simulink model "WindTurbine_TypeIV_HM"  (R2025a)
settings: Solver=FixedStepDiscrete  StartTime=0  StopTime=3  FixedStep=Ts  RelTol=1e-3  EnableMultiTasking=on
InitFcn:
  | load('xInitial_WPP.mat');
  | Ts = 50e-6;
undefined symbols (not defined in the file): D1, Delta, DiscIntNeverNeededParam, LowerLimit, magnitude, UpperLimit
libraries: powerlib x47, simulink x28, powerlib_meascontrol x17, powerlib_extras x6
(part 2 of 2)

== system WindTurbine_TypeIV_HM/Generic Type IV HM/Predictor4 ==
  in : Inport
  Delay : Delay  DelayLength=1  InitialCondition=Init_value  SampleTime=Ts
  Delay1 : Delay  DelayLength=1  InitialCondition=Init_value  SampleTime=Ts
  Gain : Gain  Gain=2
  Sum1 : Sum  Inputs=|+-
  out : Outport
  wires:
  Gain/1 -> Sum1/1
  Delay/1 -> Delay1/1, Gain/1
  Sum1/1 -> out/1
  Delay1/1 -> Sum1/2
  in/1 -> Delay/1

== system WindTurbine_TypeIV_HM/Generic Type IV HM/Predictor6 ==
  in : Inport
  Delay : Delay  DelayLength=1  InitialCondition=Init_value  SampleTime=Ts
  Delay1 : Delay  DelayLength=1  InitialCondition=Init_value  SampleTime=Ts
  Gain : Gain  Gain=2
  Sum1 : Sum  Inputs=|+-
  out : Outport
  wires:
  Gain/1 -> Sum1/1
  Delay/1 -> Delay1/1, Gain/1
  Sum1/1 -> out/1
  Delay1/1 -> Sum1/2
  in/1 -> Delay/1

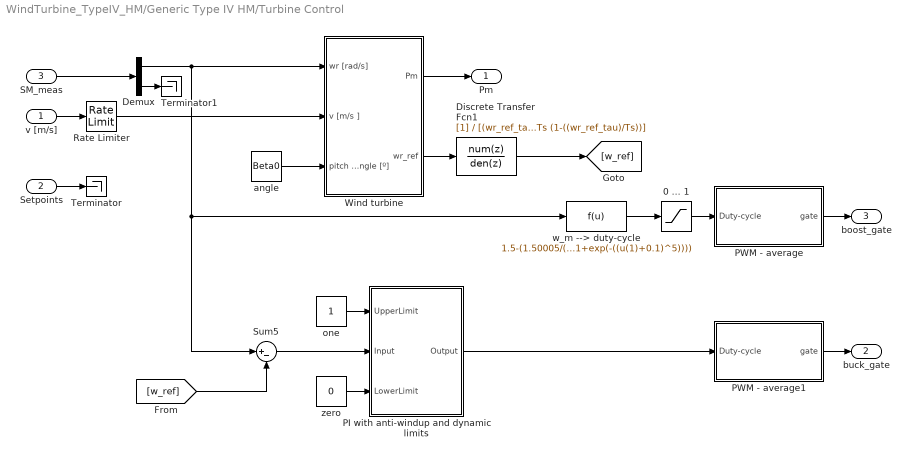
== system WindTurbine_TypeIV_HM/Generic Type IV HM/Turbine Control ==
  v [m/s] : Inport
  Setpoints : Inport  Port=2
  SM_meas : Inport  Port=3
  0 ... 1 : Saturate  UpperLimit=1  LowerLimit=0
  Demux : Demux  Outputs=2
  Discrete Transfer Fcn1 : DiscreteTransferFcn  Denominator=[(wr_ref_tau)/Ts (1-((wr_ref_tau)/Ts))]  InitialStates=w_init  SampleTime=Ts
  PI with anti-windup and dynamic limits : Subsystem  mask(Discrete PI Controller with anti-windup and dynamic limiters){Kp=Vdc1_Kp, Ki=Vdc1_Ki, Init=Vdc1_stateInit, Ts=Ts}
      mask prompts: Kp "Proportional gain (Kp):"; Ki "Integral gain (Ki):"; Init "State initial value:"; Ts "Sample time:"
      mask Display:
      | disp('PI-\nAST');
      | port_label('input',1,'UpperLimit');
      | port_label('input',2,'In');
      | port_label('input',3,'LowerLimit');
      | port_label('output',1,'Out');
  PWM - average : Subsystem  mask{fboost=f_boost, Ts=Ts}
      mask prompts: fboost "PWM frequency:"; Ts "Sample time (Ts):"
  PWM - average1 : Subsystem  mask{fboost=f_boost, Ts=Ts}
      mask prompts: fboost "PWM frequency:"; Ts "Sample time (Ts):"
  Rate Limiter : RateLimiter  RisingSlewLimit=v_rise_rate  FallingSlewLimit=v_fall_rate  SampleTimeMode=inherited  InitialCondition=v_init
  Sum5 : Sum  Inputs=|+-
  Terminator : Terminator
  Terminator1 : Terminator
  Wind turbine : Subsystem
  angle : Constant  Value=Beta0
  one : Constant
  w_m --> duty-cycle : Fcn  Expr=1.5-(1.50005/(1+exp(-((u(1)+0.1)^5))))
  zero : Constant  Value=0
  Pm : Outport
  buck_gate : Outport  Port=2
  boost_gate : Outport  Port=3
  wires:
  [w_ref] -> Sum5/2
  angle/1 -> Wind turbine/3(pitch angle [º])
  w_m --> duty-cycle/1 -> 0 ... 1/1
  0 ... 1/1 -> PWM - average/1(Duty-cycle)
  Rate Limiter/1 -> Wind turbine/2("v [m/s ] ")
  PWM - average/1(gate) -> boost_gate/1
  v [m/s]/1 -> Rate Limiter/1
  Wind turbine/1(Pm) -> Pm/1
  Wind turbine/2(wr_ref) -> Discrete Transfer Fcn1/1
  Setpoints/1 -> Terminator/1
  SM_meas/1 -> Demux/1
  Demux/1 -> w_m --> duty-cycle/1, Sum5/1, Wind turbine/1(wr [rad/s])
  Demux/2 -> Terminator1/1
  Sum5/1 -> PI with anti-windup and dynamic limits/2(Input)
  Discrete Transfer Fcn1/1 -> [w_ref]
  zero/1 -> PI with anti-windup and dynamic limits/3(LowerLimit)
  one/1 -> PI with anti-windup and dynamic limits/1(UpperLimit)
  PI with anti-windup and dynamic limits/1(Output) -> PWM - average1/1(Duty-cycle)
  PWM - average1/1(gate) -> buck_gate/1

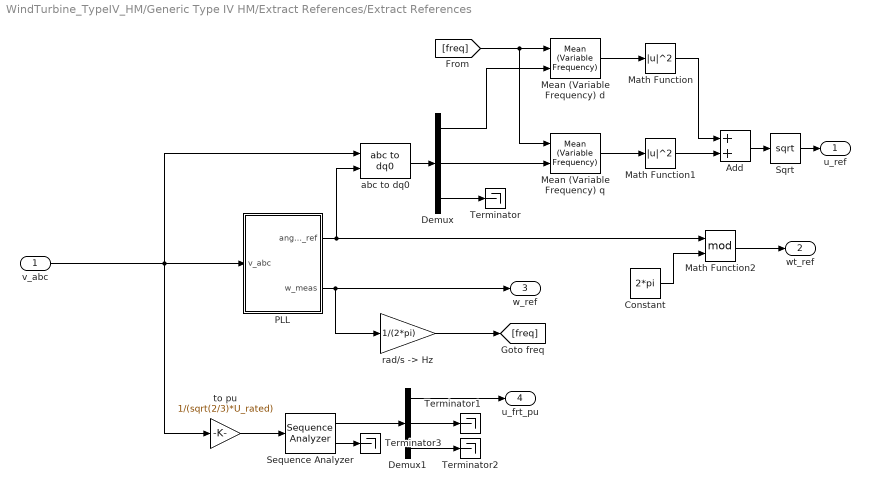
== system WindTurbine_TypeIV_HM/Generic Type IV HM/Extract References/Extract References ==
  v_abc : Inport
  Add : Sum
  Constant : Constant  Value=2*pi
  Demux : Demux  Outputs=3
  Demux1 : Demux  Outputs=3
  Math Function : Math  Operator=magnitude^2  SignedPower=on
  Math Function1 : Math  Operator=magnitude^2  SignedPower=on
  Math Function2 : Math  Operator=mod  SignedPower=on
  Mean (Variable Frequency) d : powerlib_meascontrol/Measurements/Mean (Variable Frequency)  Finit=f_rated  Fmin=0.9*f_rated  Vinit=0  Ts=Ts
  Mean (Variable Frequency) q : powerlib_meascontrol/Measurements/Mean (Variable Frequency)  Finit=f_rated  Fmin=0.9*f_rated  Vinit=0  Ts=Ts
  PLL : Subsystem
  Sequence Analyzer : powerlib_meascontrol/Measurements/Sequence Analyzer  Freq=f_rated  n=1  seq=Positive Negative Zero  InInit=[1, 0]  Ts=Ts
  Sqrt : Sqrt
  Terminator{,1..3} (4 alike) : Terminator
  abc to dq0 : powerlib_meascontrol/Transformations/abc to dq0  Alignment=90 degrees behind phase A axis
  "rad/s -> Hz" : Gain  Gain=1/(2*pi)
  to pu : Gain  Gain=1/(sqrt(2/3)*U_rated)
  u_ref : Outport
  wt_ref : Outport  Port=2
  w_ref : Outport  Port=3
  u_frt_pu : Outport  Port=4
  wires:
  abc to dq0/1 -> Demux/1
  Demux/3 -> Terminator/1
  Math Function/1 -> Add/1
  PLL/1(angle_ref) -> abc to dq0/2, Math Function2/1
  Math Function1/1 -> Add/2
  Add/1 -> Sqrt/1
  Sqrt/1 -> u_ref/1
  v_abc/1 -> PLL/1(v_abc), to pu/1, abc to dq0/1
  Sequence Analyzer/1 -> Demux1/1
  Demux1/2 -> Terminator1/1
  Demux1/3 -> Terminator2/1
  Sequence Analyzer/2 -> Terminator3/1
  Demux1/1 -> u_frt_pu/1
  [freq] -> Mean (Variable Frequency) q/1, Mean (Variable Frequency) d/1
  Mean (Variable Frequency) d/1 -> Math Function/1
  Demux/1 -> Mean (Variable Frequency) d/2
  Mean (Variable Frequency) q/1 -> Math Function1/1
  Demux/2 -> Mean (Variable Frequency) q/2
  Constant/1 -> Math Function2/2
  Math Function2/1 -> wt_ref/1
  PLL/2(w_meas) -> w_ref/1, "rad/s -> Hz"/1
  "rad/s -> Hz"/1 -> [freq]
  to pu/1 -> Sequence Analyzer/1

== system WindTurbine_TypeIV_HM/Generic Type IV HM/Extract References/Measurement Filter (Current) ==
  Meas_in : Inport
  Demux : Demux  Outputs=3
      settings: DisplayOption=none
  Discrete 2nd-Order Filter2 : powerlib_extras/Discrete  Control Blocks/Discrete  2nd-Order Filter  FilterType=Lowpass  Fo=Freq  Zeta=Zeta  Ts=Ts  Initialize=off  Vac_Init=[0.8 -25 60]  Vdc_Init=-0.4  PlotResponse=off  param1=[1 500 1]
  Discrete 2nd-Order Filter3 : powerlib_extras/Discrete  Control Blocks/Discrete  2nd-Order Filter  FilterType=Lowpass  Fo=Freq  Zeta=Zeta  Ts=Ts  Initialize=off  Vac_Init=[0.8 -25 60]  Vdc_Init=-0.4  PlotResponse=off  param1=[1 500 1]
  Discrete 2nd-Order Filter4 : powerlib_extras/Discrete  Control Blocks/Discrete  2nd-Order Filter  FilterType=Lowpass  Fo=Freq  Zeta=Zeta  Ts=Ts  Initialize=off  Vac_Init=[0.8 -25 60]  Vdc_Init=-0.4  PlotResponse=off  param1=[1 500 1]
  Mux1 : Mux  Inputs=3
  Filt_out : Outport
  wires:
  Discrete 2nd-Order Filter4/1 -> Mux1/3
  Discrete 2nd-Order Filter3/1 -> Mux1/2
  Demux/3 -> Discrete 2nd-Order Filter4/1
  Demux/1 -> Discrete 2nd-Order Filter2/1
  Meas_in/1 -> Demux/1
  Demux/2 -> Discrete 2nd-Order Filter3/1
  Discrete 2nd-Order Filter2/1 -> Mux1/1
  Mux1/1 -> Filt_out/1

== system WindTurbine_TypeIV_HM/Generic Type IV HM/Extract References/Measurement Filter (Voltage) ==
  Meas_in : Inport
  Demux : Demux  Outputs=3
      settings: DisplayOption=none
  Discrete 2nd-Order Filter2 : powerlib_extras/Discrete  Control Blocks/Discrete  2nd-Order Filter  FilterType=Lowpass  Fo=Freq  Zeta=Zeta  Ts=Ts  Initialize=off  Vac_Init=[0.8 -25 60]  Vdc_Init=-0.4  PlotResponse=off  param1=[1 500 1]
  Discrete 2nd-Order Filter3 : powerlib_extras/Discrete  Control Blocks/Discrete  2nd-Order Filter  FilterType=Lowpass  Fo=Freq  Zeta=Zeta  Ts=Ts  Initialize=off  Vac_Init=[0.8 -25 60]  Vdc_Init=-0.4  PlotResponse=off  param1=[1 500 1]
  Discrete 2nd-Order Filter4 : powerlib_extras/Discrete  Control Blocks/Discrete  2nd-Order Filter  FilterType=Lowpass  Fo=Freq  Zeta=Zeta  Ts=Ts  Initialize=off  Vac_Init=[0.8 -25 60]  Vdc_Init=-0.4  PlotResponse=off  param1=[1 500 1]
  Mux1 : Mux  Inputs=3
  Filt_out : Outport
  wires:
  Mux1/1 -> Filt_out/1
  Discrete 2nd-Order Filter2/1 -> Mux1/1
  Demux/2 -> Discrete 2nd-Order Filter3/1
  Meas_in/1 -> Demux/1
  Demux/1 -> Discrete 2nd-Order Filter2/1
  Demux/3 -> Discrete 2nd-Order Filter4/1
  Discrete 2nd-Order Filter3/1 -> Mux1/2
  Discrete 2nd-Order Filter4/1 -> Mux1/3

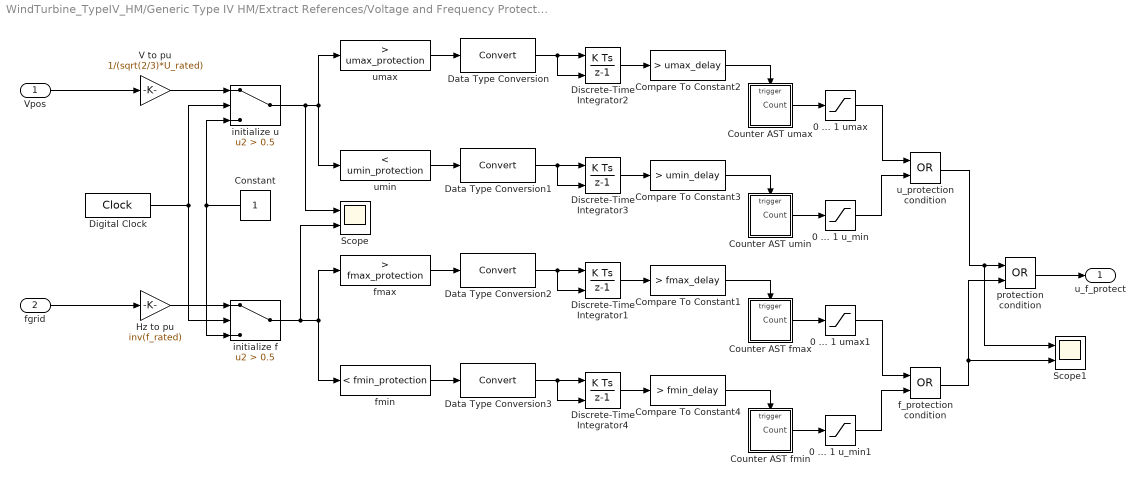
== system WindTurbine_TypeIV_HM/Generic Type IV HM/Extract References/Voltage and Frequency Protection ==
  Vpos : Inport
  fgrid : Inport  Port=2
  0 ... 1 u_min : Saturate  UpperLimit=1  LowerLimit=0
  0 ... 1 u_min1 : Saturate  UpperLimit=1  LowerLimit=0
  0 ... 1 umax : Saturate  UpperLimit=1  LowerLimit=0
  0 ... 1 umax1 : Saturate  UpperLimit=1  LowerLimit=0
  Compare To Constant1 : simulink/Logic and Bit Operations/Compare To Constant  relop=>  const=fmax_delay  OutDataTypeStr=boolean
  Compare To Constant2 : simulink/Logic and Bit Operations/Compare To Constant  relop=>  const=umax_delay  OutDataTypeStr=boolean
  Compare To Constant3 : simulink/Logic and Bit Operations/Compare To Constant  relop=>  const=umin_delay  OutDataTypeStr=boolean
  Compare To Constant4 : simulink/Logic and Bit Operations/Compare To Constant  relop=>  const=fmin_delay  OutDataTypeStr=boolean
  Constant : Constant
  Counter AST fmax : Subsystem
  Counter AST fmin : Subsystem
  Counter AST umax : Subsystem
  Counter AST umin : Subsystem
  Data Type Conversion{,1..3} (4 alike) : DataTypeConversion  SaturateOnIntegerOverflow=off  RndMeth=Floor
  Digital Clock : DigitalClock  SampleTime=Ts
  Discrete-Time Integrator{1..4} (4 alike) : DiscreteIntegrator  ExternalReset=falling  SampleTime=Ts  ICPrevOutput=DiscIntNeverNeededParam  ICPrevScaledInput=DiscIntNeverNeededParam
  Hz to pu : Gain  Gain=inv(f_rated)
  Scope : Scope  NumInputPorts=2
      settings: ActiveDisplayYMinimum=-0.20067  ActiveDisplayYMaximum=1.81542
  Scope1 : Scope  NumInputPorts=2
      settings: ActiveDisplayYMinimum=-1  ActiveDisplayYMaximum=1  DataLoggingVariableName=ScopeData2
  V to pu : Gain  Gain=1/(sqrt(2/3)*U_rated)
  f_protection condition : Logic  Operator=OR  AllPortsSameDT=off  OutDataTypeStr=boolean
  fmax : simulink/Logic and Bit Operations/Compare To Constant  relop=>  const=fmax_protection  OutDataTypeStr=boolean
  fmin : simulink/Logic and Bit Operations/Compare To Constant  relop=<  const=fmin_protection  OutDataTypeStr=boolean
  initialize f : Switch  Criteria=u2 > Threshold  Threshold=0.5  SaturateOnIntegerOverflow=off  InputSameDT=off
  initialize u : Switch  Criteria=u2 > Threshold  Threshold=0.5  SaturateOnIntegerOverflow=off  InputSameDT=off
  protection condition : Logic  Operator=OR  AllPortsSameDT=off  OutDataTypeStr=boolean
  u_protection condition : Logic  Operator=OR  AllPortsSameDT=off  OutDataTypeStr=boolean
  umax : simulink/Logic and Bit Operations/Compare To Constant  relop=>  const=umax_protection  OutDataTypeStr=boolean
  umin : simulink/Logic and Bit Operations/Compare To Constant  relop=<  const=umin_protection  OutDataTypeStr=boolean
  u_f_protect : Outport
  wires:
  Discrete-Time Integrator1/1 -> Compare To Constant1/1
  Counter AST fmin/1(Count) -> 0 ... 1 u_min1/1
  Compare To Constant4/1 -> Counter AST fmin/Trigger
  umax/1 -> Data Type Conversion/1
  0 ... 1 u_min/1 -> u_protection condition/2
  Discrete-Time Integrator3/1 -> Compare To Constant3/1
  Compare To Constant1/1 -> Counter AST fmax/Trigger
  Counter AST umin/1(Count) -> 0 ... 1 u_min/1
  fmin/1 -> Data Type Conversion3/1
  0 ... 1 umax1/1 -> f_protection condition/1
  Discrete-Time Integrator4/1 -> Compare To Constant4/1
  Counter AST fmax/1(Count) -> 0 ... 1 umax1/1
  Data Type Conversion/1 -> Discrete-Time Integrator2/2, Discrete-Time Integrator2/1
  umin/1 -> Data Type Conversion1/1
  Compare To Constant3/1 -> Counter AST umin/Trigger
  Compare To Constant2/1 -> Counter AST umax/Trigger
  fmax/1 -> Data Type Conversion2/1
  0 ... 1 u_min1/1 -> f_protection condition/2
  Data Type Conversion3/1 -> Discrete-Time Integrator4/2, Discrete-Time Integrator4/1
  Data Type Conversion2/1 -> Discrete-Time Integrator1/1, Discrete-Time Integrator1/2
  Discrete-Time Integrator2/1 -> Compare To Constant2/1
  0 ... 1 umax/1 -> u_protection condition/1
  Counter AST umax/1(Count) -> 0 ... 1 umax/1
  Data Type Conversion1/1 -> Discrete-Time Integrator3/1, Discrete-Time Integrator3/2
  fgrid/1 -> Hz to pu/1
  V to pu/1 -> initialize u/1
  Hz to pu/1 -> initialize f/1
  f_protection condition/1 -> Scope1/2, protection condition/2
  protection condition/1 -> u_f_protect/1
  Digital Clock/1 -> initialize u/2, initialize f/2
  Constant/1 -> initialize f/3, initialize u/3
  initialize u/1 -> Scope/1, umin/1, umax/1
  Vpos/1 -> V to pu/1
  u_protection condition/1 -> Scope1/1, protection condition/1
  initialize f/1 -> Scope/2, fmax/1, fmin/1

== system WindTurbine_TypeIV_HM/Generic Type IV HM/Grid-Side Inverter Control/Counter AST ==
  Trigger : TriggerPort  VariantControl=Variant  PortDimensions=1
  Constant : Constant
  Memory : Memory  InheritSampleTime=on
  Sum : Sum  Inputs=|++
  Count : Outport
  wires:
  Constant/1 -> Sum/2
  Sum/1 -> Memory/1, Count/1
  Memory/1 -> Sum/1

== system WindTurbine_TypeIV_HM/Generic Type IV HM/Grid-Side Inverter Control/FRT_ramp_p ==
  note: Aramis Schwanka Trevisan adapted from:
      | Beat Ronner
      | ABB Industrie AG
      | Turgi, Switzerland
  UpperLimit : Inport
  u : Inport  Port=2
  LowerLimit : Inport  Port=3
  Saturation : simulink/Discontinuities/Saturation Dynamic  OutMin=[]  OutMax=[]  OutDataTypeStr=Inherit: Same as second input  OutDataType=fixdt(1, 16)  OutScaling=2^-10  DoSatur=off
  Sum : Sum  Inputs=|++  InputSameDT=on  SaturateOnIntegerOverflow=on  OutDataTypeStr=Inherit: Same as first input
  Sum7 : Sum  Inputs=|+-  InputSameDT=on  SaturateOnIntegerOverflow=on  OutDataTypeStr=Inherit: Same as first input
  Unit Delay : UnitDelay  InitialCondition=1  SampleTime=Ts  HasFrameUpgradeWarning=on
  l Ts : Gain  Gain=Ts
  u Ts : Gain  Gain=Ts
  y : Outport
  wires:
  Sum7/1 -> Saturation/2
  Saturation/1 -> Sum/1
  UpperLimit/1 -> u Ts/1
  LowerLimit/1 -> l Ts/1
  Sum/1 -> Unit Delay/1, y/1  "y"
  Unit Delay/1 -> Sum/2, Sum7/2  "y-1"
  u/1 -> Sum7/1
  u Ts/1 -> Saturation/1
  l Ts/1 -> Saturation/3

== system WindTurbine_TypeIV_HM/Generic Type IV HM/Grid-Side Inverter Control/FRT_ramp_q ==
  note: Aramis Schwanka Trevisan adapted from:
      | Beat Ronner
      | ABB Industrie AG
      | Turgi, Switzerland
  UpperLimit : Inport
  u : Inport  Port=2
  LowerLimit : Inport  Port=3
  Saturation : simulink/Discontinuities/Saturation Dynamic  OutMin=[]  OutMax=[]  OutDataTypeStr=Inherit: Same as second input  OutDataType=fixdt(1, 16)  OutScaling=2^-10  DoSatur=off
  Sum : Sum  Inputs=|++  InputSameDT=on  SaturateOnIntegerOverflow=on  OutDataTypeStr=Inherit: Same as first input
  Sum7 : Sum  Inputs=|+-  InputSameDT=on  SaturateOnIntegerOverflow=on  OutDataTypeStr=Inherit: Same as first input
  Unit Delay : UnitDelay  InitialCondition=1  SampleTime=Ts  HasFrameUpgradeWarning=on
  l Ts : Gain  Gain=Ts
  u Ts : Gain  Gain=Ts
  y : Outport
  wires:
  l Ts/1 -> Saturation/3
  u Ts/1 -> Saturation/1
  u/1 -> Sum7/1
  Unit Delay/1 -> Sum7/2, Sum/2  "y-1"
  Sum/1 -> y/1, Unit Delay/1  "y"
  LowerLimit/1 -> l Ts/1
  UpperLimit/1 -> u Ts/1
  Saturation/1 -> Sum/1
  Sum7/1 -> Saturation/2

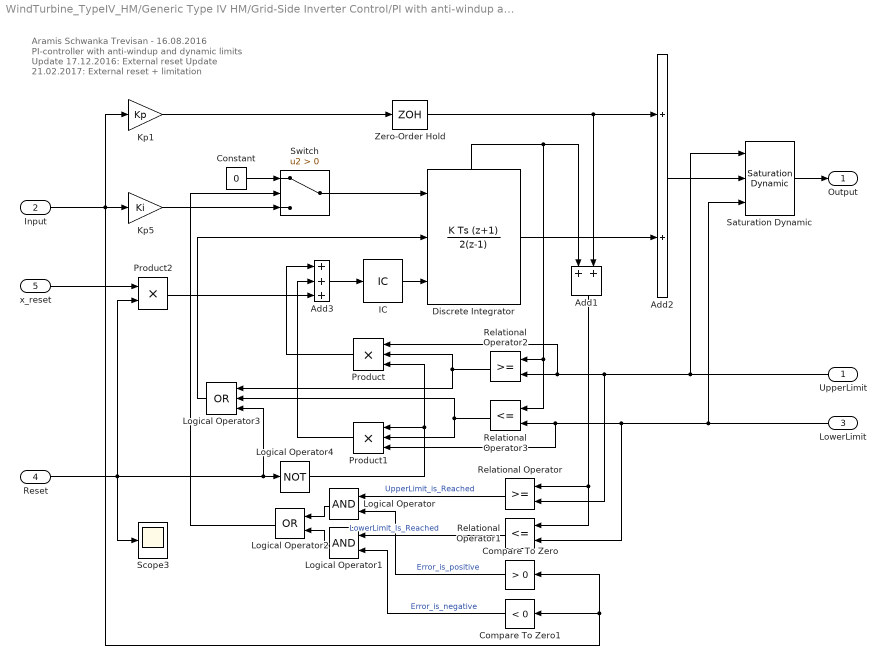
== system WindTurbine_TypeIV_HM/Generic Type IV HM/Grid-Side Inverter Control/PI with anti-windup and dynamic limits - Id ==
  note: Aramis Schwanka Trevisan - 16.08.2016
      | PI-controller with anti-windup and dynamic limits
      | Update 17.12.2016: External reset
      | Update 21.02.2017: External reset + limitation
  UpperLimit : Inport
  Input : Inport  Port=2
  LowerLimit : Inport  Port=3
  Reset : Inport  Port=4
  x_reset : Inport  Port=5
  Add1 : Sum
  Add2 : Sum
  Add3 : Sum  Inputs=+++
  Compare To Zero : simulink/Logic and Bit Operations/Compare To Zero  relop=>  OutDataTypeStr=uint8  ZeroCross=off
  Compare To Zero1 : simulink/Logic and Bit Operations/Compare To Zero  relop=<  OutDataTypeStr=uint8  ZeroCross=off
  Constant : Constant  Value=0
  Discrete Integrator : DiscreteIntegrator  IntegratorMethod=Integration: Trapezoidal  gainval=1  ExternalReset=sampled level  InitialConditionSource=external  InitialCondition=Init  SampleTime=Ts  UpperSaturationLimit=UpperLimit  LowerSaturationLimit=LowerLimit  ShowStatePort=on  ICPrevOutput=DiscIntNeverNeededParam  ICPrevScaledInput=DiscIntNeverNeededParam
  IC : InitialCondition  Value=Init
  Kp1 : Gain  Gain=Kp  SaturateOnIntegerOverflow=on  SampleTime=Ts  OutDataTypeStr=Inherit: Same as input  ParamDataTypeStr=Inherit: Same as input
  Kp5 : Gain  Gain=Ki  SaturateOnIntegerOverflow=on  SampleTime=Ts  OutDataTypeStr=Inherit: Same as input  ParamDataTypeStr=Inherit: Same as input
  Logical Operator : Logic  AllPortsSameDT=off  OutDataTypeStr=boolean
  Logical Operator1 : Logic  AllPortsSameDT=off  OutDataTypeStr=boolean
  Logical Operator2 : Logic  Operator=OR  AllPortsSameDT=off  OutDataTypeStr=boolean
  Logical Operator3 : Logic  Operator=OR  Inputs=3  AllPortsSameDT=off  OutDataTypeStr=boolean
  Logical Operator4 : Logic  Operator=NOT  Inputs=3  AllPortsSameDT=off  OutDataTypeStr=boolean
  Product : Product  Inputs=3
  Product1 : Product  Inputs=3
  Product2 : Product
  Relational Operator : RelationalOperator  OutDataTypeStr=boolean  InputSameDT=off
  Relational Operator1 : RelationalOperator  Operator=<=  OutDataTypeStr=boolean  InputSameDT=off
  Relational Operator2 : RelationalOperator  OutDataTypeStr=boolean  InputSameDT=off
  Relational Operator3 : RelationalOperator  Operator=<=  OutDataTypeStr=boolean  InputSameDT=off
  Saturation Dynamic : simulink/Discontinuities/Saturation Dynamic  OutMin=[]  OutMax=[]  OutDataTypeStr=Inherit: Same as second input  OutDataType=fixdt(1, 16)  OutScaling=2^-10  DoSatur=off
  Scope3 : Scope
      settings: ActiveDisplayYMinimum=-0.125  ActiveDisplayYMaximum=1.125
  Switch : Switch  Criteria=u2 > Threshold  SaturateOnIntegerOverflow=off  InputSameDT=off
  Zero-Order Hold : ZeroOrderHold  SampleTime=Ts
  Output : Outport
  wires:
  Reset/1 -> Scope3/1, Product2/2, Logical Operator3/3, Logical Operator4/1
  IC/1 -> Discrete Integrator/3
  Switch/1 -> Discrete Integrator/1
  Compare To Zero1/1 -> Logical Operator1/2  "Error_is_negative"
  Logical Operator/1 -> Logical Operator2/1
  Relational Operator/1 -> Logical Operator/1  "UpperLimit_is_Reached"
  Relational Operator1/1 -> Logical Operator1/1  "LowerLimit_Is_Reached"
  Saturation Dynamic/1 -> Output/1
  Logical Operator2/1 -> Switch/2
  Constant/1 -> Switch/1
  Kp5/1 -> Switch/3
  Add2/1 -> Saturation Dynamic/2
  Kp1/1 -> Zero-Order Hold/1
  Add1/1 -> Relational Operator/1, Relational Operator1/1
  Input/1 -> Kp5/1, Compare To Zero1/1, Compare To Zero/1, Kp1/1
  Compare To Zero/1 -> Logical Operator/2  "Error_is_positive"
  Logical Operator1/1 -> Logical Operator2/2
  Relational Operator2/1 -> Logical Operator3/1, Product/2
  Relational Operator3/1 -> Product1/2, Logical Operator3/2
  Logical Operator3/1 -> Discrete Integrator/2
  Add3/1 -> IC/1
  Product1/1 -> Add3/2
  UpperLimit/1 -> Saturation Dynamic/1, Relational Operator/2, Product/1, Relational Operator2/2
  Discrete Integrator/State -> Add1/1, Relational Operator3/1, Relational Operator2/1
  Discrete Integrator/1 -> Add2/2
  Logical Operator4/1 -> Product/3, Product1/1
  LowerLimit/1 -> Saturation Dynamic/3, Relational Operator1/2, Relational Operator3/2, Product1/3
  Product2/1 -> Add3/3
  Product/1 -> Add3/1
  x_reset/1 -> Product2/1
  Zero-Order Hold/1 -> Add2/1, Add1/2

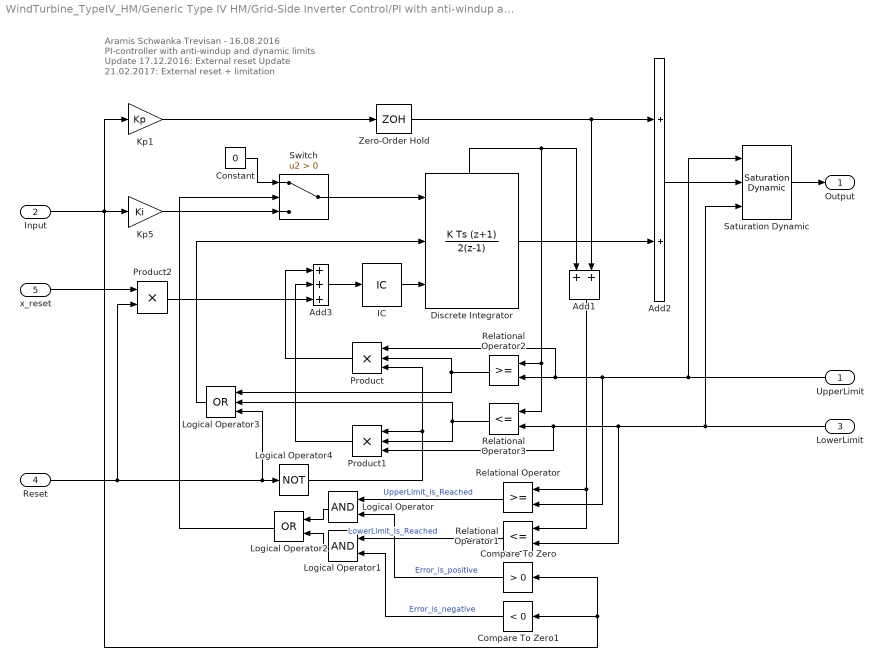
== system WindTurbine_TypeIV_HM/Generic Type IV HM/Grid-Side Inverter Control/PI with anti-windup and dynamic limits - Iq ==
  note: Aramis Schwanka Trevisan - 16.08.2016
      | PI-controller with anti-windup and dynamic limits
      | Update 17.12.2016: External reset
      | Update 21.02.2017: External reset + limitation
  UpperLimit : Inport
  Input : Inport  Port=2
  LowerLimit : Inport  Port=3
  Reset : Inport  Port=4
  x_reset : Inport  Port=5
  Add1 : Sum
  Add2 : Sum
  Add3 : Sum  Inputs=+++
  Compare To Zero : simulink/Logic and Bit Operations/Compare To Zero  relop=>  OutDataTypeStr=uint8  ZeroCross=off
  Compare To Zero1 : simulink/Logic and Bit Operations/Compare To Zero  relop=<  OutDataTypeStr=uint8  ZeroCross=off
  Constant : Constant  Value=0
  Discrete Integrator : DiscreteIntegrator  IntegratorMethod=Integration: Trapezoidal  gainval=1  ExternalReset=sampled level  InitialConditionSource=external  InitialCondition=Init  SampleTime=Ts  UpperSaturationLimit=UpperLimit  LowerSaturationLimit=LowerLimit  ShowStatePort=on  ICPrevOutput=DiscIntNeverNeededParam  ICPrevScaledInput=DiscIntNeverNeededParam
  IC : InitialCondition  Value=Init
  Kp1 : Gain  Gain=Kp  SaturateOnIntegerOverflow=on  SampleTime=Ts  OutDataTypeStr=Inherit: Same as input  ParamDataTypeStr=Inherit: Same as input
  Kp5 : Gain  Gain=Ki  SaturateOnIntegerOverflow=on  SampleTime=Ts  OutDataTypeStr=Inherit: Same as input  ParamDataTypeStr=Inherit: Same as input
  Logical Operator : Logic  AllPortsSameDT=off  OutDataTypeStr=boolean
  Logical Operator1 : Logic  AllPortsSameDT=off  OutDataTypeStr=boolean
  Logical Operator2 : Logic  Operator=OR  AllPortsSameDT=off  OutDataTypeStr=boolean
  Logical Operator3 : Logic  Operator=OR  Inputs=3  AllPortsSameDT=off  OutDataTypeStr=boolean
  Logical Operator4 : Logic  Operator=NOT  Inputs=3  AllPortsSameDT=off  OutDataTypeStr=boolean
  Product : Product  Inputs=3
  Product1 : Product  Inputs=3
  Product2 : Product
  Relational Operator : RelationalOperator  OutDataTypeStr=boolean  InputSameDT=off
  Relational Operator1 : RelationalOperator  Operator=<=  OutDataTypeStr=boolean  InputSameDT=off
  Relational Operator2 : RelationalOperator  OutDataTypeStr=boolean  InputSameDT=off
  Relational Operator3 : RelationalOperator  Operator=<=  OutDataTypeStr=boolean  InputSameDT=off
  Saturation Dynamic : simulink/Discontinuities/Saturation Dynamic  OutMin=[]  OutMax=[]  OutDataTypeStr=Inherit: Same as second input  OutDataType=fixdt(1, 16)  OutScaling=2^-10  DoSatur=off
  Switch : Switch  Criteria=u2 > Threshold  SaturateOnIntegerOverflow=off  InputSameDT=off
  Zero-Order Hold : ZeroOrderHold  SampleTime=Ts
  Output : Outport
  wires:
  Saturation Dynamic/1 -> Output/1
  Reset/1 -> Product2/2, Logical Operator3/3, Logical Operator4/1
  IC/1 -> Discrete Integrator/3
  Switch/1 -> Discrete Integrator/1
  Compare To Zero1/1 -> Logical Operator1/2  "Error_is_negative"
  Logical Operator/1 -> Logical Operator2/1
  Relational Operator/1 -> Logical Operator/1  "UpperLimit_is_Reached"
  Relational Operator1/1 -> Logical Operator1/1  "LowerLimit_Is_Reached"
  Logical Operator2/1 -> Switch/2
  Kp1/1 -> Zero-Order Hold/1
  Constant/1 -> Switch/1
  Kp5/1 -> Switch/3
  Add2/1 -> Saturation Dynamic/2
  Zero-Order Hold/1 -> Add2/1, Add1/2
  Add1/1 -> Relational Operator/1, Relational Operator1/1
  Input/1 -> Kp5/1, Compare To Zero1/1, Compare To Zero/1, Kp1/1
  Compare To Zero/1 -> Logical Operator/2  "Error_is_positive"
  Logical Operator1/1 -> Logical Operator2/2
  Relational Operator2/1 -> Logical Operator3/1, Product/2
  Relational Operator3/1 -> Product1/2, Logical Operator3/2
  Logical Operator3/1 -> Discrete Integrator/2
  Add3/1 -> IC/1
  Product1/1 -> Add3/2
  UpperLimit/1 -> Saturation Dynamic/1, Relational Operator/2, Product/1, Relational Operator2/2
  Discrete Integrator/State -> Add1/1, Relational Operator3/1, Relational Operator2/1
  Discrete Integrator/1 -> Add2/2
  Logical Operator4/1 -> Product/3, Product1/1
  LowerLimit/1 -> Saturation Dynamic/3, Relational Operator1/2, Relational Operator3/2, Product1/3
  Product2/1 -> Add3/3
  Product/1 -> Add3/1
  x_reset/1 -> Product2/1

== system WindTurbine_TypeIV_HM/Generic Type IV HM/Grid-Side Inverter Control/PWM - average ==
  note: Aramis Schwanka Trevisan
      | Adapted from: Philippe Le-Huy
  Duty-cycle : Inport
  Add : Sum  Inputs=+-
  Digital Clock : DigitalClock  SampleTime=Ts
  Divide : Product  Inputs=*/
  Mod : Math  Operator=mod  SignedPower=on
  Nb_of_samples_by_cycle : Constant  Value=1/fboost/Ts  SampleTime=Ts
  Product : Product
  Product1 : Product
  Rounding Function1 : Rounding  Operator=round
  Saturation : Saturate  UpperLimit=1  LowerLimit=0
  Ts : Constant  Value=Ts  SampleTime=Ts
  gate : Outport
  wires:
  Nb_of_samples_by_cycle/1 -> Rounding Function1/1
  Digital Clock/1 -> Mod/1
  Duty-cycle/1 -> Add/1
  Divide/1 -> Add/2
  Product/1 -> Divide/2, Mod/2
  Ts/1 -> Product/1
  Rounding Function1/1 -> Product1/2, Product/2
  Add/1 -> Product1/1
  Product1/1 -> Saturation/1
  Saturation/1 -> gate/1
  Mod/1 -> Divide/1

== system WindTurbine_TypeIV_HM/Generic Type IV HM/Grid-Side Inverter Control/Predictor1 ==
  in : Inport
  Delay : Delay  DelayLength=1  InitialCondition=Init_value  SampleTime=Ts
  Delay1 : Delay  DelayLength=1  InitialCondition=Init_value  SampleTime=Ts
  Gain : Gain  Gain=2
  Sum1 : Sum  Inputs=|+-
  out : Outport
  wires:
  in/1 -> Delay/1
  Delay1/1 -> Sum1/2
  Sum1/1 -> out/1
  Delay/1 -> Gain/1, Delay1/1
  Gain/1 -> Sum1/1

== system WindTurbine_TypeIV_HM/Generic Type IV HM/Grid-Side Inverter Control/Predictor2 ==
  in : Inport
  Delay : Delay  DelayLength=1  InitialCondition=Init_value  SampleTime=Ts
  Delay1 : Delay  DelayLength=1  InitialCondition=Init_value  SampleTime=Ts
  Gain : Gain  Gain=2
  Sum1 : Sum  Inputs=|+-
  out : Outport
  wires:
  Gain/1 -> Sum1/1
  Delay/1 -> Delay1/1, Gain/1
  Sum1/1 -> out/1
  Delay1/1 -> Sum1/2
  in/1 -> Delay/1

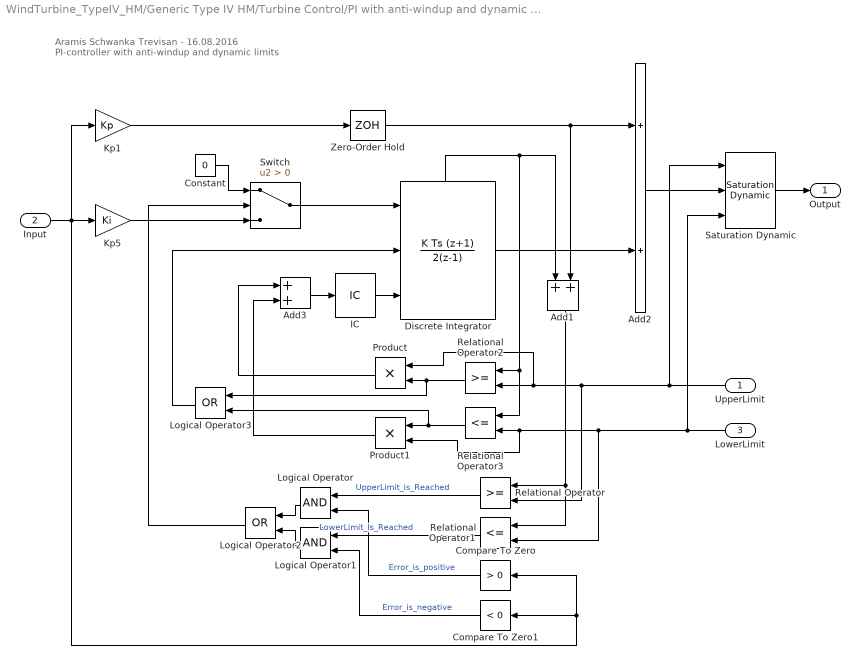
== system WindTurbine_TypeIV_HM/Generic Type IV HM/Turbine Control/PI with anti-windup and dynamic limits ==
  note: Aramis Schwanka Trevisan - 16.08.2016
      | PI-controller with anti-windup and dynamic limits
  UpperLimit : Inport
  Input : Inport  Port=2
  LowerLimit : Inport  Port=3
  Add1 : Sum
  Add2 : Sum
  Add3 : Sum
  Compare To Zero : simulink/Logic and Bit Operations/Compare To Zero  relop=>  OutDataTypeStr=uint8  ZeroCross=off
  Compare To Zero1 : simulink/Logic and Bit Operations/Compare To Zero  relop=<  OutDataTypeStr=uint8  ZeroCross=off
  Constant : Constant  Value=0
  Discrete Integrator : DiscreteIntegrator  IntegratorMethod=Integration: Trapezoidal  gainval=1  ExternalReset=sampled level  InitialConditionSource=external  InitialCondition=Init  SampleTime=Ts  UpperSaturationLimit=UpperLimit  LowerSaturationLimit=LowerLimit  ShowStatePort=on  ICPrevOutput=DiscIntNeverNeededParam  ICPrevScaledInput=DiscIntNeverNeededParam
  IC : InitialCondition  Value=Init
  Kp1 : Gain  Gain=Kp  SaturateOnIntegerOverflow=on  SampleTime=Ts  OutDataTypeStr=Inherit: Same as input  ParamDataTypeStr=Inherit: Same as input
  Kp5 : Gain  Gain=Ki  SaturateOnIntegerOverflow=on  SampleTime=Ts  OutDataTypeStr=Inherit: Same as input  ParamDataTypeStr=Inherit: Same as input
  Logical Operator : Logic  AllPortsSameDT=off  OutDataTypeStr=boolean
  Logical Operator1 : Logic  AllPortsSameDT=off  OutDataTypeStr=boolean
  Logical Operator2 : Logic  Operator=OR  AllPortsSameDT=off  OutDataTypeStr=boolean
  Logical Operator3 : Logic  Operator=OR  AllPortsSameDT=off  OutDataTypeStr=boolean
  Product : Product
  Product1 : Product
  Relational Operator : RelationalOperator  OutDataTypeStr=boolean  InputSameDT=off
  Relational Operator1 : RelationalOperator  Operator=<=  OutDataTypeStr=boolean  InputSameDT=off
  Relational Operator2 : RelationalOperator  OutDataTypeStr=boolean  InputSameDT=off
  Relational Operator3 : RelationalOperator  Operator=<=  OutDataTypeStr=boolean  InputSameDT=off
  Saturation Dynamic : simulink/Discontinuities/Saturation Dynamic  OutMin=[]  OutMax=[]  OutDataTypeStr=Inherit: Same as second input  OutDataType=fixdt(1, 16)  OutScaling=2^-10  DoSatur=off
  Switch : Switch  Criteria=u2 > Threshold  SaturateOnIntegerOverflow=off  InputSameDT=off
  Zero-Order Hold : ZeroOrderHold  SampleTime=Ts
  Output : Outport
  wires:
  Discrete Integrator/1 -> Add2/2
  Discrete Integrator/State -> Relational Operator2/1, Relational Operator3/1, Add1/1
  UpperLimit/1 -> Relational Operator2/2, Product/1, Relational Operator/2, Saturation Dynamic/1
  Product/1 -> Add3/1
  Product1/1 -> Add3/2
  Add3/1 -> IC/1
  Logical Operator3/1 -> Discrete Integrator/2
  Relational Operator3/1 -> Product1/1, Logical Operator3/2
  Relational Operator2/1 -> Product/2, Logical Operator3/1
  LowerLimit/1 -> Relational Operator3/2, Product1/2, Relational Operator1/2, Saturation Dynamic/3
  Logical Operator1/1 -> Logical Operator2/2
  Compare To Zero/1 -> Logical Operator/2  "Error_is_positive"
  Input/1 -> Kp1/1, Compare To Zero/1, Compare To Zero1/1, Kp5/1
  Add1/1 -> Relational Operator1/1, Relational Operator/1
  Zero-Order Hold/1 -> Add1/2, Add2/1
  Add2/1 -> Saturation Dynamic/2
  Kp5/1 -> Switch/3
  Constant/1 -> Switch/1
  Kp1/1 -> Zero-Order Hold/1
  Logical Operator2/1 -> Switch/2
  Saturation Dynamic/1 -> Output/1
  Relational Operator1/1 -> Logical Operator1/1  "LowerLimit_Is_Reached"
  Relational Operator/1 -> Logical Operator/1  "UpperLimit_is_Reached"
  Logical Operator/1 -> Logical Operator2/1
  Compare To Zero1/1 -> Logical Operator1/2  "Error_is_negative"
  Switch/1 -> Discrete Integrator/1
  IC/1 -> Discrete Integrator/3

== system WindTurbine_TypeIV_HM/Generic Type IV HM/Turbine Control/PWM - average ==
  Duty-cycle : Inport
  Add : Sum  Inputs=+-
  Digital Clock : DigitalClock  SampleTime=Ts
  Divide : Product  Inputs=*/
  Mod : Math  Operator=mod  SignedPower=on
  Nb_of_samples_by_cycle : Constant  Value=1/fboost/Ts  SampleTime=Ts
  Product : Product
  Product1 : Product
  Rounding Function1 : Rounding  Operator=round
  Saturation : Saturate  UpperLimit=1  LowerLimit=0
  Ts : Constant  Value=Ts  SampleTime=Ts
  gate : Outport
  wires:
  Nb_of_samples_by_cycle/1 -> Rounding Function1/1
  Digital Clock/1 -> Mod/1
  Duty-cycle/1 -> Add/1
  Divide/1 -> Add/2
  Product/1 -> Divide/2, Mod/2
  Ts/1 -> Product/1
  Rounding Function1/1 -> Product1/2, Product/2
  Add/1 -> Product1/1
  Product1/1 -> Saturation/1
  Saturation/1 -> gate/1
  Mod/1 -> Divide/1

== system WindTurbine_TypeIV_HM/Generic Type IV HM/Turbine Control/PWM - average1 ==
  Duty-cycle : Inport
  Add : Sum  Inputs=+-
  Digital Clock : DigitalClock  SampleTime=Ts
  Divide : Product  Inputs=*/
  Mod : Math  Operator=mod  SignedPower=on
  Nb_of_samples_by_cycle : Constant  Value=1/fboost/Ts  SampleTime=Ts
  Product : Product
  Product1 : Product
  Rounding Function1 : Rounding  Operator=round
  Saturation : Saturate  UpperLimit=1  LowerLimit=0
  Ts : Constant  Value=Ts  SampleTime=Ts
  gate : Outport
  wires:
  Mod/1 -> Divide/1
  Saturation/1 -> gate/1
  Product1/1 -> Saturation/1
  Add/1 -> Product1/1
  Rounding Function1/1 -> Product/2, Product1/2
  Ts/1 -> Product/1
  Product/1 -> Mod/2, Divide/2
  Divide/1 -> Add/2
  Duty-cycle/1 -> Add/1
  Digital Clock/1 -> Mod/1
  Nb_of_samples_by_cycle/1 -> Rounding Function1/1

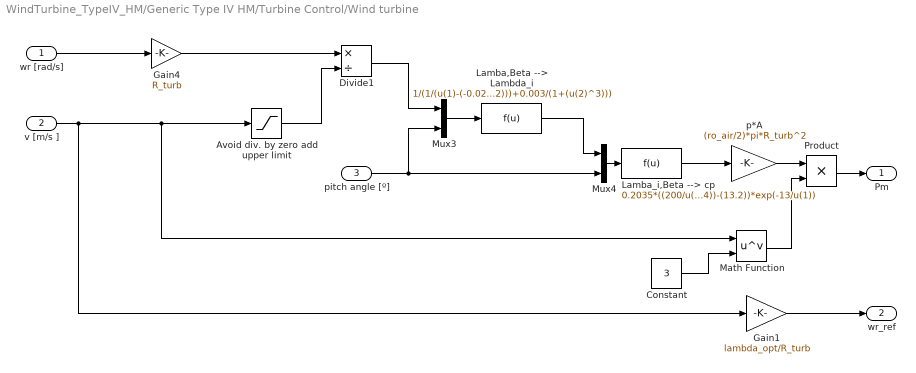
== system WindTurbine_TypeIV_HM/Generic Type IV HM/Turbine Control/Wind turbine ==
  wr [rad/s] : Inport
  "v [m/s ] " : Inport  Port=2
  pitch angle [º] : Inport  Port=3
  Avoid div. by zero add upper limit : Saturate  UpperLimit=vspeed_max  LowerLimit=vspeed_min
  Constant : Constant  Value=3
  Divide1 : Product  Inputs=*/
  Gain1 : Gain  Gain=lambda_opt/R_turb
  Gain4 : Gain  Gain=R_turb
  Lamba,Beta --> Lambda_i : Fcn  Expr=1/(1/(u(1)-(-0.02*u(2)))+0.003/(1+(u(2)^3)))
  Lamba_i,Beta --> cp : Fcn  Expr=0.2035*((200/u(1))-(0.15*u(2))-(0.05*(u(2)^2.14))-(13.2))*exp(-13/u(1))
  Math Function : Math  Operator=pow  SignedPower=on
  Mux3 : Mux  Inputs=2
  Mux4 : Mux  Inputs=2
  Product : Product
  p*A : Gain  Gain=(ro_air/2)*pi*R_turb^2
  Pm : Outport
  wr_ref : Outport  Port=2
  wires:
  Avoid div. by zero add upper limit/1 -> Divide1/2
  Gain4/1 -> Divide1/1
  Mux3/1 -> Lamba,Beta --> Lambda_i/1
  Lamba,Beta --> Lambda_i/1 -> Mux4/1
  Divide1/1 -> Mux3/1
  Mux4/1 -> Lamba_i,Beta --> cp/1
  pitch angle [º]/1 -> Mux4/2, Mux3/2
  Lamba_i,Beta --> cp/1 -> p*A/1
  Constant/1 -> Math Function/2
  p*A/1 -> Product/1
  Math Function/1 -> Product/2
  Product/1 -> Pm/1
  wr [rad/s]/1 -> Gain4/1
  "v [m/s ] "/1 -> Avoid div. by zero add upper limit/1, Math Function/1, Gain1/1
  Gain1/1 -> wr_ref/1

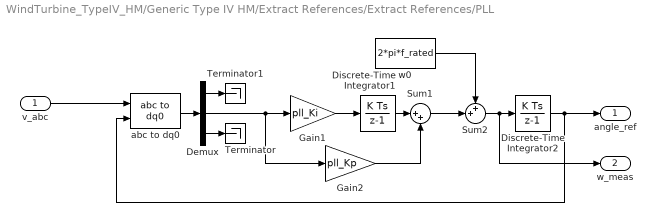
== system WindTurbine_TypeIV_HM/Generic Type IV HM/Extract References/Extract References/PLL ==
  v_abc : Inport
  Demux : Demux  Outputs=3
  Discrete-Time Integrator1 : DiscreteIntegrator  SampleTime=Ts  ICPrevOutput=DiscIntNeverNeededParam  ICPrevScaledInput=DiscIntNeverNeededParam
  Discrete-Time Integrator2 : DiscreteIntegrator  InitialCondition=2*pi*f_rated  SampleTime=Ts  ICPrevOutput=DiscIntNeverNeededParam  ICPrevScaledInput=DiscIntNeverNeededParam
  Gain1 : Gain  Gain=pll_Ki
  Gain2 : Gain  Gain=pll_Kp
  Sum1 : Sum  Inputs=|++
  Sum2 : Sum  Inputs=++|
  Terminator : Terminator
  Terminator1 : Terminator
  abc to dq0 : powerlib_meascontrol/Transformations/abc to dq0  Alignment=90 degrees behind phase A axis
  w0 : Constant  Value=2*pi*f_rated
  angle_ref : Outport
  w_meas : Outport  Port=2
  wires:
  w0/1 -> Sum2/1
  Sum2/1 -> w_meas/1, Discrete-Time Integrator2/1
  Demux/3 -> Terminator/1
  abc to dq0/1 -> Demux/1
  v_abc/1 -> abc to dq0/1
  Demux/2 -> Gain2/1, Gain1/1
  Gain2/1 -> Sum1/2
  Gain1/1 -> Discrete-Time Integrator1/1
  Discrete-Time Integrator1/1 -> Sum1/1
  Discrete-Time Integrator2/1 -> angle_ref/1, abc to dq0/2
  Sum1/1 -> Sum2/2
  Demux/1 -> Terminator1/1

== system WindTurbine_TypeIV_HM/Generic Type IV HM/Extract References/Voltage and Frequency Protection/Counter AST fmax ==
  Trigger : TriggerPort  VariantControl=Variant  PortDimensions=1
  Constant : Constant
  Memory : Memory  InheritSampleTime=on
  Sum : Sum  Inputs=|++
  Count : Outport
  wires:
  Memory/1 -> Sum/1
  Sum/1 -> Count/1, Memory/1
  Constant/1 -> Sum/2

== system WindTurbine_TypeIV_HM/Generic Type IV HM/Extract References/Voltage and Frequency Protection/Counter AST fmin ==
  Trigger : TriggerPort  VariantControl=Variant  PortDimensions=1
  Constant : Constant
  Memory : Memory  InheritSampleTime=on
  Sum : Sum  Inputs=|++
  Count : Outport
  wires:
  Constant/1 -> Sum/2
  Sum/1 -> Memory/1, Count/1
  Memory/1 -> Sum/1

== system WindTurbine_TypeIV_HM/Generic Type IV HM/Extract References/Voltage and Frequency Protection/Counter AST umax ==
  Trigger : TriggerPort  VariantControl=Variant  PortDimensions=1
  Constant : Constant
  Memory : Memory  InheritSampleTime=on
  Sum : Sum  Inputs=|++
  Count : Outport
  wires:
  Constant/1 -> Sum/2
  Sum/1 -> Memory/1, Count/1
  Memory/1 -> Sum/1

== system WindTurbine_TypeIV_HM/Generic Type IV HM/Extract References/Voltage and Frequency Protection/Counter AST umin ==
  Trigger : TriggerPort  VariantControl=Variant  PortDimensions=1
  Constant : Constant
  Memory : Memory  InheritSampleTime=on
  Sum : Sum  Inputs=|++
  Count : Outport
  wires:
  Memory/1 -> Sum/1
  Sum/1 -> Count/1, Memory/1
  Constant/1 -> Sum/2
